simulink model "BLDC"  (R2025a)
settings: Solver=VariableStepAuto  StartTime=0.0  StopTime=1  RelTol=1e-3
undefined symbols (not defined in the file): Ion, Lithium
libraries: spsMosfetLib x6, spsSeriesRLCBranchLib x2, spsBatteryLib x1, slpidlib x1, spsPermanentMagnetSynchronousMachineLib x1, sps_lib x1
settings Model: Creator=saswa  LastModifiedBy=saswa

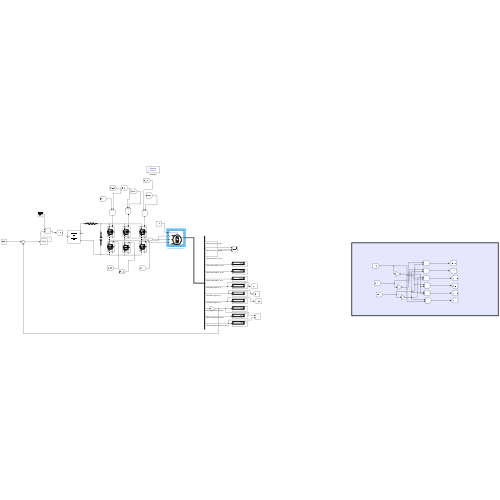
[thumbnail: Simulink's stored preview of the top-level diagram]
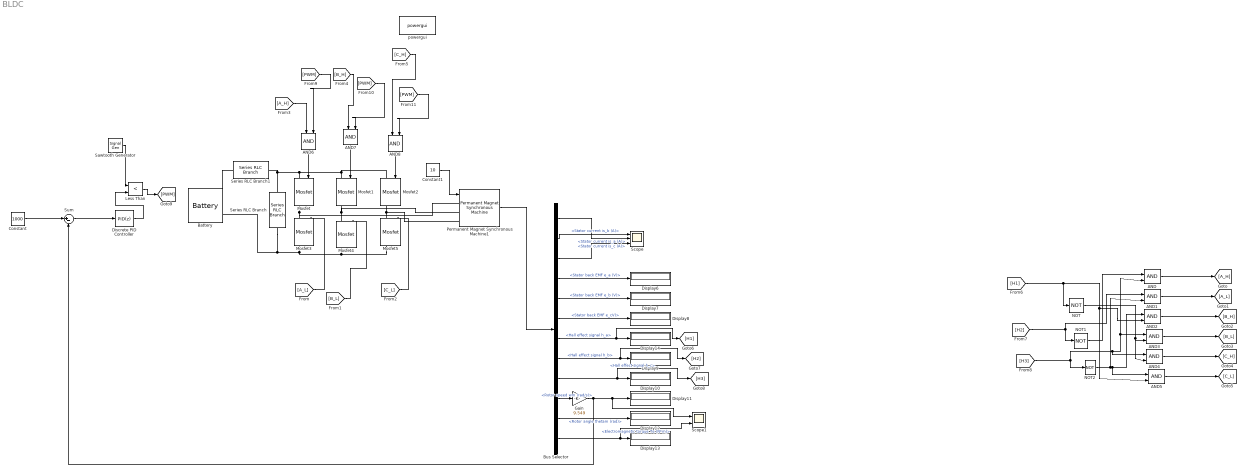
== system BLDC ==
  AND{,1..8} (9 alike) : Logic  IconShape=distinctive  AllPortsSameDT=off  OutDataTypeStr=boolean
  Battery : spsBatteryLib/Battery  BatType=Lithium-Ion  NomV=200  NomQ=5.4  SOC=100  Batt_Tr=30  PresetModel=on  MaxQ=5.4  MinV=150  FullV=232.7974  Dis_rate=2.3478  R=0.37037  Normal_OP=4.8835  expZone="[216.0772     0.2653043]"
  Bus Selector : BusSelector  OutputSignals=Stator current is_a (A),Stator current is_b (A),Stator current is_c (A),Stator back EMF e_a (V),Stator back EMF e_b (V),Stator back EMF e_cV),Hall effect signal h_a,Hall effect signal h_b,Hall effect signal h_c,Rotor speed wm (rad/s),Rotor angle thetam (rad),Electromagnetic torque Te (N*m)
  Constant : Constant  Value=1000
  Constant1 : Constant  Value=10
  Discrete PID Controller : slpidlib/PID Controller  Controller=PID  Form=Parallel  TimeDomain=Discrete-time  UseExternalTs=off  SampleTime=-1  IntegratorMethod=Forward Euler  FilterMethod=Forward Euler  ControllerParametersSource=internal  P=0.1  I=2  UseKiTs=off  D=0  UseExternalDerivativeSource=off  N=100  UseFilter=on  TunerSelectOption=Transfer Function Based (PID Tuner App)  InitialConditionSource=internal  InitialConditionForIntegrator=0  InitialConditionForFilter=0  DifferentiatorICPrevScaledInput=0  ExternalReset=none  TrackingMode=off  Kt=1  LimitOutput=off  SatLimitsSource=internal  UpperSaturationLimit=inf  LowerSaturationLimit=-inf  LinearizeAsGain=off  AntiWindupMode=none  Kb=1  LimitIntegrator=off  UpperIntegratorSaturationLimit=inf  LowerIntegratorSaturationLimit=-inf  POutMin=[]  POutMax=[]  IOutMin=[]  IOutMax=[]  DOutMin=[]  DOutMax=[]  NOutMin=[]  NOutMax=[]  SumOutMin=[]  SumOutMax=[]  SaturationOutMin=[]  SaturationOutMax=[]  PParamMin=[]  PParamMax=[]  IParamMin=[]  IParamMax=[]  DParamMin=[]  DParamMax=[]  NParamMin=[]  NParamMax=[]  KbParamMin=[]  KbParamMax=[]  KtParamMin=[]  KtParamMax=[]  KbOutMin=[]  KbOutMax=[]  KtOutMin=[]  KtOutMax=[]  IntegratorOutMin=[]  IntegratorOutMax=[]  FilterOutMin=[]  FilterOutMax=[]  SumI1OutMin=[]  SumI1OutMax=[]  SumI2OutMin=[]  SumI2OutMax=[]  SumI3OutMin=[]  SumI3OutMax=[]  SumI4OutMin=[]  SumI4OutMax=[]  SumDOutMin=[]  SumDOutMax=[]  DifferentiatorOutMin=[]  DifferentiatorOutMax=[]  FilterDiffOutCoefMin=[]  FilterDiffOutCoefMax=[]  ReciprocalOutMin=[]  ReciprocalOutMax=[]  SumDenOutMin=[]  SumDenOutMax=[]  SumNumOutMin=[]  SumNumOutMax=[]  DivideOutMin=[]  DivideOutMax=[]  UdiffTsProdOutMin=[]  UdiffTsProdOutMax=[]  NTsProdOutMin=[]  NTsProdOutMax=[]  UintegralTsProdOutMin=[]  UintegralTsProdOutMax=[]  UngainTsProdOutMin=[]  UngainTsProdOutMax=[]  ClampingZeroOutDataTypeStr=Inherit: Inherit via back propagation  ClampingZeroOutMin=[]  ClampingZeroOutMax=[]  FilterDenConstantOutDataTypeStr=Inherit: Inherit via back propagation  FilterDenConstantOutMin=[]  FilterDenConstantOutMax=[]  PCopyOutDataTypeStr=Inherit: Inherit via back propagation  PCopyOutMin=[]  PCopyOutMax=[]  NCopyOutDataTypeStr=Inherit: Inherit via back propagation  NCopyOutMin=[]  NCopyOutMax=[]  IntegratorContinuousStateAttributes=''  IntegratorStateMustResolveToSignalObject=off  IntegratorRTWStateStorageClass=Auto  FilterContinuousStateAttributes=''  FilterStateMustResolveToSignalObject=off  FilterRTWStateStorageClass=Auto  ParallelPVariant=InternalParameters  IdealPVariant=Disabled  IVariant=InternalParameters  DVariant=InternalParameters  IntegratorVariant=Discrete  SatVariant=Disabled  AWVariant=Passthrough  PCopyVariant=Disabled  TRVariant=Disabled  FdbkBlocksVariant=Forward  IdealPFdbkVariant=Disabled  SatFdbkVariant=Disabled  DerivativeFilterVariant=ForwardEulerFilter  NVariant=InternalParameters  NCopyVariant=Disabled  FilterICVariant=InternalICsFilter  IntegratorICVariant=InternalICs  ExternalResetVariant=Disabled  TRSumVariant=Passthrough  SumFdbkVariant=Disabled  SumVariant=Sum_PID  TsampFilterVariant=InternalTs  TsampNgainVariant=Passthrough  TsampIntegralVariant=Disabled_SignalSpec  ExternalSaturationOutDataTypeStr=Inherit: Same as second input  DerivativeSourceVariant=ErrorSignal  PreIntVariant=InternalPreInt
      settings: LibrarySourceBlock=simulink/Discrete/Discrete PID Controller
  Display{6..14} (9 alike) : Display
  Gain : Gain  Gain=9.549
  Less Than : RelationalOperator  Operator=<  OutDataTypeStr=boolean  RndMeth=Simplest  InputSameDT=off
  Mosfet{,1..5} (6 alike) : spsMosfetLib/Mosfet  Ron=0.1  Lon=0  Rd=0.01  Vfd=0  IC=0  Rs=1e5  Cs=inf  Measurements=on
  NOT : Logic  Operator=NOT  IconShape=distinctive  AllPortsSameDT=off  OutDataTypeStr=boolean
  NOT1 : Logic  Operator=NOT  IconShape=distinctive  AllPortsSameDT=off  OutDataTypeStr=boolean
  NOT2 : Logic  Operator=NOT  IconShape=distinctive  AllPortsSameDT=off  OutDataTypeStr=boolean
  Permanent Magnet Synchronous Machine1 : spsPermanentMagnetSynchronousMachineLib/Permanent Magnet Synchronous Machine  NbPhases=3  FluxDistribution=Trapezoidal  RotorType=Round  MechanicalLoad=Torque Tm  PresetModel="15:  87.75 Nm 560 Vdc 3000 RPM - 97.96 Nm"  ShowDetailedParameters=on  MeasurementBus=off  Resistance=0.05  Inductance=8.5e-3  dqInductances=[8.5e-3,8.5e-3]  La=0.000795  MachineConstant=Flux linkage established by magnets (V.s)  Flux=0.192  VoltageCst=160.8495  TorqueCst=1.536  Flat=120  Mechanical=[0.011 0.001417 4 0]  PolePairs=4  InitialConditions=[0,0, 0,0]  InitialConditions5ph=[0 0 0 0 0 0]  RefAngle=90 degrees behind phase A axis (modified Park)  IterativeDiscreteModel=Trapezoidal non iterative  TsBlock=-1  TsPowergui=0
  Sawtooth Generator : SignalGenerator  WaveForm=sawtooth  Frequency=10000  Units=rad/sec
  Scope : Scope  NumInputPorts=3
      settings: ActiveDisplayYMinimum=-68.128525857337877  ActiveDisplayYMaximum=68.129258006119258
  Scope1 : Scope  NumInputPorts=2
      settings: ActiveDisplayYMinimum=-248.09829101295696  ActiveDisplayYMaximum=1507.3761567259889
  Series RLC Branch : spsSeriesRLCBranchLib/Series RLC Branch  LConnTagsString=__new0  RConnTagsString=__new0  BranchType=C  Resistance=1  Inductance=1e-3  SetiL0=off  InitialCurrent=0  Capacitance=1e-3  Setx0=off  InitialVoltage=0  Measurements=None
  Series RLC Branch1 : spsSeriesRLCBranchLib/Series RLC Branch  LConnTagsString=__new0  RConnTagsString=__new0  BranchType=R  Resistance=5  Inductance=1e-3  SetiL0=off  InitialCurrent=0  Capacitance=1e-6  Setx0=off  InitialVoltage=0  Measurements=None
  Sum : Sum  Inputs=|+-
  powergui : sps_lib/powergui  Priority=1  SimulationMode=Discrete  SampleTime=1e-6  frequency=60  Iterations=50  frequencyindice=0  Pbase=100e6  ErrMax=1e-4  UnitsV=kV  UnitsW=MW  buscounter=0  FunctionMessages=off  echomessages=off  EnableUseOfTLC=off  CurrentSourceSwitches=off  DisableSnubberDevices=off  DisableRonSwitches=off  DisableVfSwitches=off  DisplayEquations=off  AutomaticDiscreteSolvers=off  SolverType=Tustin/Backward Euler (TBE)  Interpol=off  ExternalGateDelay=off  methode=off  Ts=100  x0status=blocks  SPID=on  SwTol=0  HookPort=off  NonlinearTolerance=1e-4  nMaxIteration=100  ContinueOnMaxIteration=off  RestoreLinks=warning  ResistiveCurrentMeasurement=off  Frange=[0:2:500]  Ylog=off  Xlog=on  ShowGrid=off  save=off  variable=ZData  structure=0  ZoomFFT=off  StartTime=0.0  cycles=1  DisplayStyle=1  fundamental=60  FreqAxis=off  MaxFrequency=1000  frequencyindicesteady=1  RmsSteady=1  display=off
  wires:
  AND/1 -> [A_H]
  AND1/1 -> [A_L]
  AND2/1 -> [B_H]
  AND3/1 -> [B_L]
  AND4/1 -> [C_H]
  AND5/1 -> [C_L]
  [H1] -> NOT/1, AND2/2, AND5/2
  [H2] -> AND1/1, NOT1/1
  [H3] -> AND4/1, AND3/1, AND/2, NOT2/1
  NOT1/1 -> AND/1
  NOT2/1 -> AND2/1, AND5/1, AND1/2
  NOT/1 -> AND3/2, AND4/2
  [A_L] -> Mosfet3/1
  [B_L] -> Mosfet4/1
  [C_L] -> Mosfet5/1
  Permanent Magnet Synchronous Machine1/1 -> Bus Selector/1
  Bus Selector/1 -> Scope/2  "<Stator current is_a (A)>"
  Bus Selector/2 -> Scope/1  "<Stator current is_b (A)>"
  Bus Selector/3 -> Scope/3  "<Stator current is_c (A)>"
  Bus Selector/4 -> Display6/1  "<Stator back EMF e_a (V)>"
  Bus Selector/5 -> Display7/1  "<Stator back EMF e_b (V)>"
  Bus Selector/6 -> Display8/1  "<Stator back EMF e_cV)>"
  Bus Selector/8 -> [H2], Display9/1  "<Hall effect signal h_b>"
  Bus Selector/9 -> [H3], Display10/1  "<Hall effect signal h_c>"
  Bus Selector/11 -> Display12/1  "<Rotor angle thetam (rad)>"
  Bus Selector/12 -> Scope1/2, Display13/1  "<Electromagnetic torque Te (N*m)>"
  Bus Selector/7 -> [H1], Display14/1  "<Hall effect signal h_a>"
  [A_H] -> AND6/1
  AND6/1 -> Mosfet/1
  Constant/1 -> Sum/1
  Sum/1 -> Discrete PID Controller/1
  [B_H] -> AND7/1
  [C_H] -> AND8/1
  AND8/1 -> Mosfet2/1
  Constant1/1 -> Permanent Magnet Synchronous Machine1/1
  Discrete PID Controller/1 -> Less Than/2
  Sawtooth Generator/1 -> Less Than/1
  Less Than/1 -> [PWM]
  AND7/1 -> Mosfet1/1
  Bus Selector/10 -> Gain/1  "<Rotor speed wm (rad/s)>"
  [PWM] -> AND6/2
  [PWM] -> AND7/2
  [PWM] -> AND8/2
  Gain/1 -> Sum/2, Scope1/1, Display11/1
  connections:
  Mosfet/RConn1 -- Permanent Magnet Synchronous Machine1/LConn1 -- Mosfet3/LConn1
  Mosfet1/RConn1 -- Mosfet4/LConn1 -- Permanent Magnet Synchronous Machine1/LConn2
  Mosfet2/RConn1 -- Permanent Magnet Synchronous Machine1/LConn3 -- Mosfet5/LConn1
  Series RLC Branch1/LConn1 -- Battery/LConn1
  Mosfet5/RConn1 -- Series RLC Branch/RConn1 -- Battery/LConn2 -- Mosfet3/RConn1 -- Mosfet4/RConn1
  Mosfet1/LConn1 -- Mosfet2/LConn1 -- Series RLC Branch/LConn1 -- Series RLC Branch1/RConn1 -- Mosfet/LConn1
